simulink model "bh_test_sfun_model"  (R2016a)
settings: Solver=FixedStepDiscrete  StartTime=0.0  StopTime=333  RelTol=1e-3
libraries: simulink_extras x2
settings Model: ExtModeTrigMode=oneshot  ExtModeArmWhenConnect=off  ExtModeAutoUpdateStatusClock=off  Creator=The MathWorks, Inc.  LastModifiedBy=bhorton
settings DataIOCC: SaveFormat=Array
settings OptimizationCC: BooleanDataType=off  ExpressionDepthLimit=2147483647  InitFltsAndDblsToZero=on
settings DebuggingCC: SaveWithParameterizedLinksMsg=none  UnderspecifiedInitializationDetection=Classic  MergeDetectMultiDrivingBlocksExec=none  SignalResolutionControl=TryResolveAllWithWarning  MultiTaskDSMMsg=warning  MultiTaskCondExecSysMsg=none  FcnCallInpInsideContextMsg=UseLocalSettings  StateNameClashWarn=warning
settings HardwareCC: ProdBitPerPointer=32  ProdLargestAtomicFloat=None  ProdIntDivRoundTo=Undefined  ProdEndianess=Unspecified  ProdWordSize=32  ProdHWDeviceType=32-bit Generic  TargetUnknown=on
settings ModelReferenceCC: PropagateSignalLabelsOutOfModel=off
settings GRTTargetCC: TargetFcnLib=ansi_tfl_tmw.mat  CombineOutputUpdateFcns=off  GRTInterface=on
settings ConfigComp: CovModelRefEnable=Off

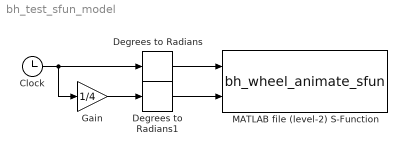
== system bh_test_sfun_model ==
  Clock : Clock
  Degrees to Radians : simulink_extras/Transformations/Degrees to Radians
  Degrees to Radians1 : simulink_extras/Transformations/Degrees to Radians
  Gain : Gain  Gain=1/4
  MATLAB file (level-2) S-Function : M-S-Function  FunctionName=bh_wheel_animate_sfun  Parameters=1, 0.3, 0.1
  wires:
  Clock/1 -> Gain/1, Degrees to Radians/1
  Degrees to Radians/1 -> MATLAB file (level-2) S-Function/1
  Degrees to Radians1/1 -> MATLAB file (level-2) S-Function/2
  Gain/1 -> Degrees to Radians1/1
